simulink library "IPT_lib"  (Simulink 7.4)
settings: Solver=ode45  StartTime=0.0  StopTime=10.0  RelTol=1e-3
values from neighbouring files (symbols this model uses):
  IPTa_i_ShuntCur = mpt.Parameter    [IPT_ANALOG_CAL.m]
  IPTc_Gain_KL30 = mpt.Parameter    [IPT_ANALOG_CAL.m]
  IPTc_Gain_MSDVolt = mpt.Parameter    [IPT_ANALOG_CAL.m]
  IPTc_Gain_PCBTemp = mpt.Parameter    [IPT_ANALOG_CAL.m]
  IPTc_Gain_PosCtrVoltRef1_back = mpt.Parameter    [IPT_ANALOG_CAL.m]
  IPTc_Gain_PosCtrVoltRef1_front = mpt.Parameter    [IPT_ANALOG_CAL.m]
  IPTc_Gain_PosCtrVoltRef2_back = mpt.Parameter    [IPT_ANALOG_CAL.m]
  IPTc_Gain_PosCtrVoltRef2_front = mpt.Parameter    [IPT_ANALOG_CAL.m]
  IPTc_pct_CellInitSoc = mpt.Parameter    [IPT_INTERNAL_CAL.m]
  IPTc_t_BMUInitTemp = mpt.Parameter    [IPT_CAN_CAL.m]
  IPTc_t_MdlInitTemp = mpt.Parameter    [IPT_CAN_CAL.m]
  IPTc_t_PCBTemp_max = mpt.Parameter    [IPT_ANALOG_CAL.m]
  IPTc_t_PCBTemp_min = mpt.Parameter    [IPT_ANALOG_CAL.m]
  IPTc_v_KL30_max = mpt.Parameter    [IPT_ANALOG_CAL.m]
  IPTc_v_KL30_min = mpt.Parameter    [IPT_ANALOG_CAL.m]
  IPTc_v_MSDVolt_max = mpt.Parameter    [IPT_ANALOG_CAL.m]
  IPTc_v_MSDVolt_min = mpt.Parameter    [IPT_ANALOG_CAL.m]
  IPTc_v_PosCtrVoltRef1_back_max = mpt.Parameter    [IPT_ANALOG_CAL.m]
  IPTc_v_PosCtrVoltRef1_back_min = mpt.Parameter    [IPT_ANALOG_CAL.m]
  IPTc_v_PosCtrVoltRef1_front_max = mpt.Parameter    [IPT_ANALOG_CAL.m]
  IPTc_v_PosCtrVoltRef1_front_min = mpt.Parameter    [IPT_ANALOG_CAL.m]
  IPTc_v_PosCtrVoltRef2_back_max = mpt.Parameter    [IPT_ANALOG_CAL.m]
  IPTc_v_PosCtrVoltRef2_back_min = mpt.Parameter    [IPT_ANALOG_CAL.m]
  IPTc_v_PosCtrVoltRef2_front_max = mpt.Parameter    [IPT_ANALOG_CAL.m]
  IPTc_v_PosCtrVoltRef2_front_min = mpt.Parameter    [IPT_ANALOG_CAL.m]
  IPTf_fac_ShuntCurCorrect = mpt.Parameter    [IPT_ANALOG_CAL.m]
undefined symbols (not defined in the file or in its folder): CTC_DriveOnline_St, CTC_FastChaOnline_St, CTC_SlowChaOnline_St, IPTa_v_PCBTemp, IPTc_Gain_BMUPowSplyCur, IPTc_Gain_ShuntCur, IPTc_Gain_USample, IPTc_i_BMUPowSplyCur_max, IPTc_i_BMUPowSplyCur_min, IPTc_i_ShuntCur_max, IPTc_i_ShuntCur_min, IPTc_v_CC2_OffDnLimit, IPTc_v_CC2_OffUpLimit, IPTc_v_CC2_OnDnLimit, IPTc_v_CC2_OnUpLimit, IPTc_v_CellInitVolt, IPTc_v_SlowChalineCnctStLowLimFir, IPTc_v_SlowChalineCnctStLowLimSec, IPTc_v_SlowChalineCnctStUppLimFir, IPTc_v_SlowChalineCnctStUppLimSec, IPTc_v_SlowChalineOpenLowLim, IPTc_v_SlowChalineOpenUppLim, IPTc_v_USample_max, IPTc_v_USample_min, IPTf_t_PCBTemp, PACK_Const_BMUNumOfPack
libraries: Defined_Functionality x129
(part 3 of 3)

== system IPT_lib/IPT/ip_digitial/ChaWake ==
  HLd_adc_ChaWake : Inport  OutDataType=fixdt(1, 16)  OutScaling=2^0
  ADC to Actual Value2 : Defined_Functionality/ADC to Actual Value  SystemSampleTime=-1  gain=0.0134277  offset=0
      settings: AttributesFormatString=[GAIN=%<gain>]\n[OFFSET=%<offset>]
  LPF : Defined_Functionality/LPF  SystemSampleTime=-1  filter_gain=0.09
      settings: AttributesFormatString=[FILTER_GAIN=%<filter_gain>]
  hysteresis1 : Defined_Functionality/hysteresis  SystemSampleTime=-1  upper_limit=IPTc_v_ChaWake_HysisUpLimit  lower_limit=IPTc_v_ChaWake_HysisDnLimit
      settings: AttributesFormatString=[UPPER_LIMIT=%<upper_limit>]\n[LOWER_LIMIT=%<lower_limit>]
  signal_debug : Defined_Functionality/signal_debug  SystemSampleTime=-1  debug_switch=IPTc_dbgsw_ChaWake  debug_value=IPTc_dbgval_ChaWake
      settings: AttributesFormatString=[SWITCH=%<debug_switch>]\n[VALUE=%<debug_value>]
  IPTd_flg_ChaWake : Outport  OutDataType=fixdt(1, 16)  OutScaling=2^0
  wires:
  hysteresis1/1 -> signal_debug/1
  ADC to Actual Value2/1 -> LPF/1
  HLd_adc_ChaWake/1 -> ADC to Actual Value2/1
  signal_debug/1 -> IPTd_flg_ChaWake/1  "IPTd_flg_ChaWake"
  LPF/1 -> hysteresis1/1

== system IPT_lib/IPT/ip_digitial/HVILSt ==
  HLd_flg_HVILSt : Inport  OutDataType=fixdt(1, 16)  OutScaling=2^0
  debounce : Defined_Functionality/debounce  SystemSampleTime=-1  debounce_time=30
      settings: AttributesFormatString=[DEBOUNCE_TIME=%<debounce_time>]
  signal_debug : Defined_Functionality/signal_debug  SystemSampleTime=-1  debug_switch=IPTc_dbgsw_HVILSt  debug_value=IPTc_dbgval_HVILSt
      settings: AttributesFormatString=[SWITCH=%<debug_switch>]\n[VALUE=%<debug_value>]
  IPTd_flg_HVILSt : Outport  OutDataType=fixdt(1, 16)  OutScaling=2^0
  wires:
  debounce/1 -> signal_debug/1
  HLd_flg_HVILSt/1 -> debounce/1
  signal_debug/1 -> IPTd_flg_HVILSt/1  "IPTd_flg_HVILSt"

== system IPT_lib/IPT/ip_digitial/KL15 ==
  HLd_adc_KL15 : Inport  OutDataType=fixdt(1, 16)  OutScaling=2^0
  ADC to Actual Value3 : Defined_Functionality/ADC to Actual Value  SystemSampleTime=-1  gain=0.0134277  offset=0
      settings: AttributesFormatString=[GAIN=%<gain>]\n[OFFSET=%<offset>]
  LPF : Defined_Functionality/LPF  SystemSampleTime=-1  filter_gain=IPTc_flter_KL15
      settings: AttributesFormatString=[FILTER_GAIN=%<filter_gain>]
  hysteresis : Defined_Functionality/hysteresis  SystemSampleTime=-1  upper_limit=IPTc_v_KL15_HysisUpLimit  lower_limit=IPTc_v_KL15_HysisDnLimit
      settings: AttributesFormatString=[UPPER_LIMIT=%<upper_limit>]\n[LOWER_LIMIT=%<lower_limit>]
  signal_debug : Defined_Functionality/signal_debug  SystemSampleTime=-1  debug_switch=IPTc_dbgsw_KL15  debug_value=IPTc_dbgval_KL15
      settings: AttributesFormatString=[SWITCH=%<debug_switch>]\n[VALUE=%<debug_value>]
  IPTd_flg_KL15 : Outport  OutDataType=fixdt(1, 16)  OutScaling=2^0
  wires:
  LPF/1 -> hysteresis/1  "IPTd_v_KL15"
  ADC to Actual Value3/1 -> LPF/1
  HLd_adc_KL15/1 -> ADC to Actual Value3/1
  signal_debug/1 -> IPTd_flg_KL15/1  "IPTd_flg_KL15"
  hysteresis/1 -> signal_debug/1

== system IPT_lib/IPT/ip_digitial/ServiceSt ==
  HLd_flg_ServSt : Inport  OutDataType=fixdt(1, 16)  OutScaling=2^0
  debounce : Defined_Functionality/debounce  SystemSampleTime=-1  debounce_time=30
      settings: AttributesFormatString=[DEBOUNCE_TIME=%<debounce_time>]
  signal_debug : Defined_Functionality/signal_debug  SystemSampleTime=-1  debug_switch=IPTc_dbgsw_ServSt  debug_value=IPTc_dbgval_ServSt
      settings: AttributesFormatString=[SWITCH=%<debug_switch>]\n[VALUE=%<debug_value>]
  IPTd_flg_ServSt : Outport  OutDataType=fixdt(1, 16)  OutScaling=2^0
  wires:
  signal_debug/1 -> IPTd_flg_ServSt/1  "IPTd_flg_ServSt"
  HLd_flg_ServSt/1 -> debounce/1
  debounce/1 -> signal_debug/1

== system IPT_lib/IPT/InternalOutputOfPlatform/RestoreMdlSoc/CellSoc ==
  CellMdlIn : Inport
  Assignment : Assignment  IndexOptions=Index vector (port)  Indices=1  OutputSizes=1
  CAN to Actual Value : Defined_Functionality/CAN to Actual Value  SystemSampleTime=-1  gain=0.01  offset=0
      settings: AttributesFormatString=[GAIN=%<gain>]\n[OFFSET=%<offset>]
  Constant2 : Constant  Value=IPTc_pct_CellInitSoc
  For Iterator : ForIterator  IterationLimit=PACK_Const_MdlNumOfPack  IterationVariableDataType=int16
  Selector : Selector  InputPortWidth=PACK_Const_MdlNumOfPack  IndexOptions=Index vector (port)  Indices=[1 3]  OutputSizes=1
  CellMdlOut : Outport  DataType=single  OutDataTypeStr=single
  wires:
  Selector/1 -> CAN to Actual Value/1
  CellMdlIn/1 -> Selector/1
  For Iterator/1 -> Selector/2, Assignment/3
  Constant2/1 -> Assignment/1
  Assignment/1 -> CellMdlOut/1
  CAN to Actual Value/1 -> Assignment/2

== system IPT_lib/IPT/ip_analog/PCBTemp/Conversion ==
  ADC : Inport  OutDataType=fixdt(1, 16)  OutScaling=2^0
  ADC to Actual Value1 : Defined_Functionality/ADC to Actual Value1  SystemSampleTime=-1  offset=IPTc_Offset_PCBTemp  gain=IPTc_Gain_PCBTemp
      settings: AttributesFormatString=[OFFSET=%<offset>]\n[GAIN=%<gain>]
  Lookup Table : Lookup  InputValues=IPTa_v_PCBTemp  Table=IPTf_t_PCBTemp  OutDataType=fixdt(1, 16)  OutScaling=2^0
  Volt : Outport  OutDataType=fixdt(1, 16)  OutScaling=2^0
  wires:
  Lookup Table/1 -> Volt/1  "IPTd_t_PCBTemp_raw"
  ADC to Actual Value1/1 -> Lookup Table/1
  ADC/1 -> ADC to Actual Value1/1

== system IPT_lib/IPT/ip_can/BMU_BMS_200ms/ErrorCode ==
  In : Inport
  Assignment : Assignment  IndexOptions=Index vector (port)  Indices=1  OutputSizes=1
  Constant2 : Constant  Value=zeros(1,PACK_Const_BMUNumOfPack)  OutDataTypeMode=uint16  OutDataTypeStr=uint16
  For Iterator : ForIterator  IterationLimit=PACK_Const_BMUNumOfPack  IterationVariableDataType=int16
  Selector : Selector  InputPortWidth=PACK_Const_BMUNumOfPack  IndexOptions=Index vector (port)  Indices=[1 3]  OutputSizes=1
  Out : Outport
  wires:
  Assignment/1 -> Out/1
  Constant2/1 -> Assignment/1
  For Iterator/1 -> Assignment/3, Selector/2
  In/1 -> Selector/1
  Selector/1 -> Assignment/2

== system IPT_lib/IPT/ip_can/BMU_BMS_200ms/NmStatus ==
  In : Inport
  Assignment : Assignment  IndexOptions=Index vector (port)  Indices=1  OutputSizes=1
  Constant2 : Constant  Value=zeros(1,PACK_Const_BMUNumOfPack)  OutDataTypeMode=uint8  OutDataTypeStr=uint8
  For Iterator : ForIterator  IterationLimit=PACK_Const_BMUNumOfPack  IterationVariableDataType=int16
  Selector : Selector  InputPortWidth=PACK_Const_BMUNumOfPack  IndexOptions=Index vector (port)  Indices=[1 3]  OutputSizes=1
  Out : Outport
  wires:
  Selector/1 -> Assignment/2
  In/1 -> Selector/1
  For Iterator/1 -> Selector/2, Assignment/3
  Constant2/1 -> Assignment/1
  Assignment/1 -> Out/1

== system IPT_lib/IPT/ip_can/BMU_BMS_200ms/NodeStatus ==
  In : Inport
  Assignment : Assignment  IndexOptions=Index vector (port)  Indices=1  OutputSizes=1
  Constant2 : Constant  Value=zeros(1,PACK_Const_BMUNumOfPack)  OutDataTypeMode=uint8  OutDataTypeStr=uint8
  For Iterator : ForIterator  IterationLimit=PACK_Const_BMUNumOfPack  IterationVariableDataType=int16
  Selector : Selector  InputPortWidth=PACK_Const_BMUNumOfPack  IndexOptions=Index vector (port)  Indices=[1 3]  OutputSizes=1
  Out : Outport
  wires:
  Assignment/1 -> Out/1
  Constant2/1 -> Assignment/1
  For Iterator/1 -> Assignment/3, Selector/2
  In/1 -> Selector/1
  Selector/1 -> Assignment/2

== system IPT_lib/IPT/ip_can/BMU_BMS_300ms/CellVolt ==
  In : Inport
  Assignment : Assignment  IndexOptions=Index vector (port)  Indices=1  OutputSizes=1
  CAN to Actual Value : Defined_Functionality/CAN to Actual Value  SystemSampleTime=-1  gain=0.001  offset=0
      settings: AttributesFormatString=[GAIN=%<gain>]\n[OFFSET=%<offset>]
  Constant2 : Constant  Value=IPTc_v_CellInitVolt
  For Iterator : ForIterator  IterationLimit=PACK_Const_CellNumOfPack  IterationVariableDataType=int16
  LPF : Defined_Functionality/LPF  SystemSampleTime=-1  filter_gain=IPTc_flter_CellVolt
      settings: AttributesFormatString=[FILTER_GAIN=%<filter_gain>]
  Selector : Selector  InputPortWidth=PACK_Const_CellNumOfPack  IndexOptions=Index vector (port)  Indices=[1 3]  OutputSizes=1
  Out : Outport
  wires:
  LPF/1 -> Assignment/2
  Selector/1 -> CAN to Actual Value/1
  In/1 -> Selector/1
  For Iterator/1 -> Assignment/3, Selector/2
  Constant2/1 -> Assignment/1
  Assignment/1 -> Out/1
  CAN to Actual Value/1 -> LPF/1

== system IPT_lib/IPT/ip_can/BMU_BMS_500ms/BMUTemp ==
  In : Inport
  Assignment : Assignment  IndexOptions=Index vector (port)  Indices=1  OutputSizes=1
  CAN to Actual Value : Defined_Functionality/CAN to Actual Value  SystemSampleTime=-1  gain=1  offset=-40
      settings: AttributesFormatString=[GAIN=%<gain>]\n[OFFSET=%<offset>]
  Constant2 : Constant  Value=IPTc_t_BMUInitTemp  OutDataTypeMode=single  OutDataTypeStr=single
  For Iterator : ForIterator  IterationLimit=PACK_Const_BMUTempSnrNumOfPack  IterationVariableDataType=int16
  LPF : Defined_Functionality/LPF  SystemSampleTime=-1  filter_gain=IPTc_flter_BMUTemp
      settings: AttributesFormatString=[FILTER_GAIN=%<filter_gain>]
  Selector : Selector  InputPortWidth=PACK_Const_BMUTempSnrNumOfPack  IndexOptions=Index vector (port)  Indices=[1 3]  OutputSizes=1
  Out : Outport
  wires:
  LPF/1 -> Assignment/2
  In/1 -> Selector/1
  For Iterator/1 -> Selector/2, Assignment/3
  Constant2/1 -> Assignment/1
  Assignment/1 -> Out/1
  Selector/1 -> CAN to Actual Value/1
  CAN to Actual Value/1 -> LPF/1

== system IPT_lib/IPT/ip_can/BMU_BMS_500ms/MdlTemp ==
  In : Inport
  Assignment : Assignment  IndexOptions=Index vector (port)  Indices=1  OutputSizes=1
  CAN to Actual Value : Defined_Functionality/CAN to Actual Value  SystemSampleTime=-1  gain=0.125  offset=-40
      settings: AttributesFormatString=[GAIN=%<gain>]\n[OFFSET=%<offset>]
  Constant2 : Constant  Value=IPTc_t_MdlInitTemp  OutDataTypeMode=single  OutDataTypeStr=single
  For Iterator : ForIterator  IterationLimit=PACK_Const_MdlTempSnrNumOfPack  IterationVariableDataType=int16
  LPF : Defined_Functionality/LPF  SystemSampleTime=-1  filter_gain=IPTc_flter_MdlTemp
      settings: AttributesFormatString=[FILTER_GAIN=%<filter_gain>]
  Selector : Selector  InputPortWidth=PACK_Const_MdlTempSnrNumOfPack  IndexOptions=Index vector (port)  Indices=[1 3]  OutputSizes=1
  Out : Outport
  wires:
  LPF/1 -> Assignment/2
  CAN to Actual Value/1 -> LPF/1
  Selector/1 -> CAN to Actual Value/1
  Assignment/1 -> Out/1
  Constant2/1 -> Assignment/1
  For Iterator/1 -> Assignment/3, Selector/2
  In/1 -> Selector/1

== system IPT_lib/IPT/ip_can/Diagnositc_Enabling/CAN_Bus_Monitoring ==
  HLd_flg_CANBusOff : Inport
  Gain : Gain  OutDataTypeStr=Inherit: Inherit via back propagation
  debounce : Defined_Functionality/debounce  SystemSampleTime=-1  debounce_time=IPTc_tm_CANBusOffDeb
      settings: AttributesFormatString=[DEBOUNCE_TIME=%<debounce_time>]
  IPTd_iflt_CANBusOff_fault : Outport
  IPTd_cflt_CANBusOff_fault : Outport  Port=2
  wires:
  debounce/1 -> IPTd_cflt_CANBusOff_fault/1
  Gain/1 -> debounce/1, IPTd_iflt_CANBusOff_fault/1
  HLd_flg_CANBusOff/1 -> Gain/1

== system IPT_lib/IPT/ip_can/Diagnositc_Enabling/CAN_Diag_Enabling ==
  IPTd_iflt_CANBusOff_fault : Inport
  IPTd_cflt_CANBusOff_fault : Inport  Port=2
  IPTd_flg_KL15 : Inport  Port=3
  Logical Operator : Logic  Inputs=3  AllPortsSameDT=off  OutDataTypeMode=boolean  LogicDataType=fixdt(0, 8)  OutDataTypeStr=boolean
  Logical Operator2 : Logic  Operator=NOT  Inputs=1  AllPortsSameDT=off  OutDataTypeMode=boolean  OutDataTypeStr=boolean
  Logical Operator3 : Logic  Operator=NOT  Inputs=1  AllPortsSameDT=off  OutDataTypeMode=boolean  OutDataTypeStr=boolean
  rising_delay : Defined_Functionality/rising_delay  SystemSampleTime=-1  delay_time=500
      settings: AttributesFormatString=[DELAY_TIME=%<delay_time>]
  signal_debug : Defined_Functionality/signal_debug  SystemSampleTime=-1  debug_switch=IPTc_dbgsw_CANDiagEnable  debug_value=IPTc_dbgval_CANDiagEnable
      settings: AttributesFormatString=[SWITCH=%<debug_switch>]\n[VALUE=%<debug_value>]
  IPTd_flg_CANDiagEnable : Outport
  wires:
  signal_debug/1 -> IPTd_flg_CANDiagEnable/1  "IPTd_flg_CANDiagEnable"
  Logical Operator/1 -> signal_debug/1
  Logical Operator3/1 -> Logical Operator/2
  IPTd_cflt_CANBusOff_fault/1 -> Logical Operator3/1
  rising_delay/1 -> Logical Operator/3
  Logical Operator2/1 -> Logical Operator/1
  IPTd_flg_KL15/1 -> rising_delay/1
  IPTd_iflt_CANBusOff_fault/1 -> Logical Operator2/1

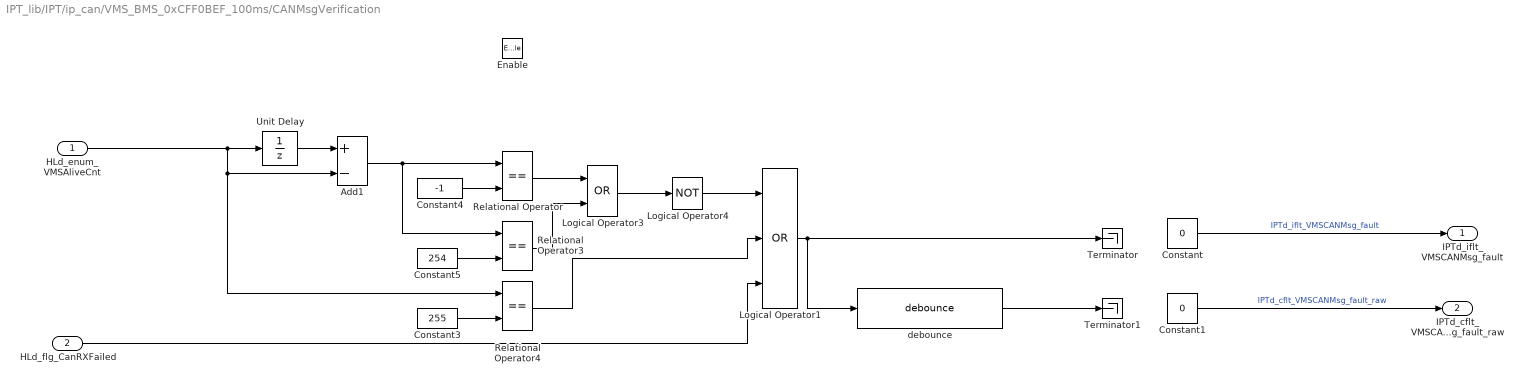
== system IPT_lib/IPT/ip_can/VMS_BMS_0xCFF0BEF_100ms/CANMsgVerification ==
  HLd_enum_VMSAliveCnt : Inport
  HLd_flg_CanRXFailed : Inport  Port=2  OutDataType=fixdt(1, 16)  OutScaling=2^0
  Enable : EnablePort
  Add1 : Sum  Inputs=+-  OutDataTypeMode=int16  OutDataTypeStr=int16
  Constant : Constant  Value=0  OutDataTypeMode=boolean  OutDataType=fixdt(1, 16)  OutScaling=2^0  OutDataTypeStr=boolean
  Constant1 : Constant  Value=0  OutDataTypeMode=boolean  OutDataType=fixdt(1, 16)  OutScaling=2^0  OutDataTypeStr=boolean
  Constant3 : Constant  Value=255  OutDataTypeMode=uint8  OutDataTypeStr=uint8
  Constant4 : Constant  Value=-1  OutDataTypeMode=int8  OutDataTypeStr=int8
  Constant5 : Constant  Value=254  OutDataTypeMode=uint8  OutDataTypeStr=uint8
  Logical Operator1 : Logic  Operator=OR  Inputs=3  AllPortsSameDT=off  OutDataTypeMode=boolean  LogicDataType=fixdt(0, 8)  OutDataTypeStr=boolean
  Logical Operator3 : Logic  Operator=OR  AllPortsSameDT=off  OutDataTypeMode=boolean  LogicDataType=fixdt(0, 8)  OutDataTypeStr=boolean
  Logical Operator4 : Logic  Operator=NOT  AllPortsSameDT=off  OutDataTypeMode=boolean  LogicDataType=fixdt(0, 8)  OutDataTypeStr=boolean
  Relational Operator : RelationalOperator  Operator===  LogicOutDataTypeMode=boolean  OutDataTypeStr=boolean
  Relational Operator3 : RelationalOperator  Operator===  LogicOutDataTypeMode=boolean  OutDataTypeStr=boolean
  Relational Operator4 : RelationalOperator  Operator===  LogicOutDataTypeMode=boolean  OutDataTypeStr=boolean
  Terminator : Terminator
  Terminator1 : Terminator
  Unit Delay : UnitDelay  SampleTime=-1
  debounce : Defined_Functionality/debounce  SystemSampleTime=-1  debounce_time=IPTc_tm_VMSCanFltDeb
      settings: AttributesFormatString=[DEBOUNCE_TIME=%<debounce_time>]
  IPTd_iflt_VMSCANMsg_fault : Outport  InitialOutput=0
  IPTd_cflt_VMSCANMsg_fault_raw : Outport  Port=2  InitialOutput=0
  wires:
  Constant1/1 -> IPTd_cflt_VMSCANMsg_fault_raw/1  "IPTd_cflt_VMSCANMsg_fault_raw"
  Constant/1 -> IPTd_iflt_VMSCANMsg_fault/1  "IPTd_iflt_VMSCANMsg_fault"
  Logical Operator3/1 -> Logical Operator4/1
  Relational Operator4/1 -> Logical Operator1/2
  Constant3/1 -> Relational Operator4/2
  Relational Operator3/1 -> Logical Operator3/2
  Relational Operator/1 -> Logical Operator3/1
  Add1/1 -> Relational Operator3/1, Relational Operator/1
  Unit Delay/1 -> Add1/1
  Constant4/1 -> Relational Operator/2
  Constant5/1 -> Relational Operator3/2
  HLd_enum_VMSAliveCnt/1 -> Relational Operator4/1, Add1/2, Unit Delay/1
  Logical Operator4/1 -> Logical Operator1/1
  Logical Operator1/1 -> Terminator/1, debounce/1
  HLd_flg_CanRXFailed/1 -> Logical Operator1/3
  debounce/1 -> Terminator1/1

== system IPT_lib/IPT/ip_can/VMS_BMS_0xCFF0BEF_100ms/HVCnctCmd ==
  HLd_flg_VehHVCnctCmd : Inport
  IPTd_iflt_VMSCANMsg_fault : Inport  Port=2
  IPTd_cflt_VMSCANMsg_fault_raw : Inport  Port=3
  Constant : Constant  Value=0  OutDataTypeMode=boolean  OutDataType=fixdt(1, 16)  OutScaling=2^0  OutDataTypeStr=boolean
  Logical Operator : Logic  Operator=NOT  AllPortsSameDT=off  OutDataTypeMode=boolean  LogicDataType=fixdt(0, 8)  OutDataTypeStr=boolean
  Switch : Switch  Criteria=u2 > Threshold  OutDataType=fixdt(1, 16)  OutScaling=2^0
  Switch2 : Switch  Criteria=u2 > Threshold  OutDataType=fixdt(1, 16)  OutScaling=2^0
  Unit Delay : UnitDelay  SampleTime=-1
  signal_debug : Defined_Functionality/signal_debug  SystemSampleTime=-1  debug_switch=IPTc_dbgsw_VehHVCnctCmd  debug_value=IPTc_dbgval_VehHVCnctCmd
      settings: AttributesFormatString=[SWITCH=%<debug_switch>]\n[VALUE=%<debug_value>]
  IPTd_flg_VehHVCnctCmd : Outport
  wires:
  IPTd_iflt_VMSCANMsg_fault/1 -> Switch2/2
  IPTd_cflt_VMSCANMsg_fault_raw/1 -> Logical Operator/1
  HLd_flg_VehHVCnctCmd/1 -> [HLd_flg_VehHVCnctCmd], Unit Delay/1
  Constant/1 -> Switch/3
  Switch2/1 -> Switch/1
  [HLd_flg_VehHVCnctCmd] -> Switch2/3
  Unit Delay/1 -> Switch2/1
  Logical Operator/1 -> Switch/2
  Switch/1 -> signal_debug/1
  signal_debug/1 -> IPTd_flg_VehHVCnctCmd/1  "IPTd_flg_VehHVCnctCmd"

== system IPT_lib/IPT/ip_can/VMS_BMS_0xCFF0BEF_100ms/KeySt ==
  HLd_enum_KeySt : Inport
  IPTd_cflt_VMSCANMsg_fault_raw : Inport  Port=2
  Constant : Constant  Value=0  OutDataTypeMode=uint8  OutDataType=fixdt(1, 16)  OutScaling=2^0  OutDataTypeStr=uint8
  Constant1 : Constant  Value=3  OutDataTypeMode=uint8  OutDataType=fixdt(1, 16)  OutScaling=2^0  OutDataTypeStr=uint8
  Gain : Gain  ParameterDataType=fixdt(1, 16)  ParameterScaling=2^0  OutDataType=fixdt(1, 16)  OutScaling=2^0  OutDataTypeStr=Inherit: Same as input
  Logical Operator : Logic  Operator=NOT  AllPortsSameDT=off  OutDataTypeMode=boolean  LogicDataType=fixdt(0, 8)  OutDataTypeStr=boolean
  Logical Operator2 : Logic  Operator=OR  AllPortsSameDT=off  OutDataTypeMode=boolean  LogicDataType=fixdt(0, 8)  OutDataTypeStr=boolean
  Relational Operator : RelationalOperator  Operator=>  LogicOutDataTypeMode=boolean  LogicDataType=fixdt(0, 8)  OutDataTypeStr=boolean
  Switch : Switch  Criteria=u2 > Threshold  OutDataType=fixdt(1, 16)  OutScaling=2^0
  Switch2 : Switch  Criteria=u2 > Threshold  OutDataType=fixdt(1, 16)  OutScaling=2^0
  Unit Delay : UnitDelay  SampleTime=-1
  debounce : Defined_Functionality/debounce  SystemSampleTime=-1  debounce_time=IPTc_tm_VMSCanFltDeb
      settings: AttributesFormatString=[DEBOUNCE_TIME=%<debounce_time>]
  signal_debug : Defined_Functionality/signal_debug  SystemSampleTime=-1  debug_switch=0  debug_value=1
      settings: AttributesFormatString=[SWITCH=%<debug_switch>]\n[VALUE=%<debug_value>]
  IPTd_enum_KeySt : Outport
  wires:
  Gain/1 -> [IPTd_enum_KeyStRaw]
  Relational Operator/1 -> Logical Operator2/1
  Logical Operator2/1 -> Switch2/2, debounce/1  "IPTd_iflt_CANBus"
  Constant1/1 -> Relational Operator/2
  IPTd_cflt_VMSCANMsg_fault_raw/1 -> Logical Operator2/2
  [IPTd_enum_KeyStRaw] -> Switch2/3
  debounce/1 -> Logical Operator/1
  HLd_enum_KeySt/1 -> Gain/1, Unit Delay/1, Relational Operator/1
  Switch/1 -> signal_debug/1
  Unit Delay/1 -> Switch2/1
  Switch2/1 -> Switch/1
  Constant/1 -> Switch/3
  Logical Operator/1 -> Switch/2
  signal_debug/1 -> IPTd_enum_KeySt/1  "IPTd_enum_KeySt"

== system IPT_lib/IPT/ip_can/VMS_BMS_0xCFF0BEF_100ms/VMSChaAllowed ==
  HLd_flg_VMSChaAllowed : Inport  DataType=boolean  OutDataTypeStr=boolean
  IPTd_iflt_CANMsg_fault : Inport  Port=2
  IPTd_cflt_VMSCANMsg_fault_raw : Inport  Port=3
  Constant : Constant  Value=0  OutDataTypeMode=boolean  OutDataType=fixdt(1, 16)  OutScaling=2^0  OutDataTypeStr=boolean
  Logical Operator : Logic  Operator=NOT  AllPortsSameDT=off  OutDataTypeMode=boolean  LogicDataType=fixdt(0, 8)  OutDataTypeStr=boolean
  Switch : Switch  Criteria=u2 > Threshold  OutDataType=fixdt(1, 16)  OutScaling=2^0
  Switch2 : Switch  Criteria=u2 > Threshold  OutDataType=fixdt(1, 16)  OutScaling=2^0
  Unit Delay1 : UnitDelay  SampleTime=-1
  debounce : Defined_Functionality/debounce  SystemSampleTime=-1  debounce_time=IPTc_tm_VMSChaAllowedDeb
      settings: AttributesFormatString=[DEBOUNCE_TIME=%<debounce_time>]
  signal_debug1 : Defined_Functionality/signal_debug  SystemSampleTime=-1  debug_switch=IPTc_dbgsw_VMSChaAllowed  debug_value=IPTc_dbgval_VMSChaAllowed
      settings: AttributesFormatString=[SWITCH=%<debug_switch>]\n[VALUE=%<debug_value>]
  IPTd_flg_VMSChaAllowed : Outport
  wires:
  debounce/1 -> signal_debug1/1
  IPTd_iflt_CANMsg_fault/1 -> Switch2/2
  IPTd_cflt_VMSCANMsg_fault_raw/1 -> Logical Operator/1
  HLd_flg_VMSChaAllowed/1 -> [HLd_flg_VMSChaAllowed], Unit Delay1/1
  Unit Delay1/1 -> Switch2/1
  [HLd_flg_VMSChaAllowed] -> Switch2/3
  Switch2/1 -> Switch/1
  Logical Operator/1 -> Switch/2
  Switch/1 -> debounce/1
  Constant/1 -> Switch/3
  signal_debug1/1 -> IPTd_flg_VMSChaAllowed/1  "IPTd_flg_VMSChaAllowed"

== system IPT_lib/IPT/ip_can/VMS_BMS_0xCFF0BEF_100ms/VMSChaStopCmd ==
  HLd_flg_VMSChaStopCmd : Inport  DataType=boolean  OutDataTypeStr=boolean
  IPTd_iflt_CANMsg_fault : Inport  Port=2
  IPTd_cflt_VMSCANMsg_fault_raw : Inport  Port=3
  Constant : Constant  OutDataTypeMode=boolean  OutDataType=fixdt(1, 16)  OutScaling=2^0  OutDataTypeStr=boolean
  Logical Operator : Logic  Operator=NOT  AllPortsSameDT=off  OutDataTypeMode=boolean  LogicDataType=fixdt(0, 8)  OutDataTypeStr=boolean
  Switch : Switch  Criteria=u2 > Threshold  OutDataType=fixdt(1, 16)  OutScaling=2^0
  Switch1 : Switch  Criteria=u2 > Threshold  OutDataType=fixdt(1, 16)  OutScaling=2^0
  Unit Delay : UnitDelay  SampleTime=-1
  debounce : Defined_Functionality/debounce  SystemSampleTime=-1  debounce_time=IPTc_tm_VMSChaStopCmdDeb
      settings: AttributesFormatString=[DEBOUNCE_TIME=%<debounce_time>]
  signal_debug : Defined_Functionality/signal_debug  SystemSampleTime=-1  debug_switch=IPTc_dbgsw_VMSChaStopCmd  debug_value=IPTc_dbgval_VMSChaStopCmd
      settings: AttributesFormatString=[SWITCH=%<debug_switch>]\n[VALUE=%<debug_value>]
  IPTd_flg_VMSChaStopCmd : Outport
  wires:
  HLd_flg_VMSChaStopCmd/1 -> [HLd_flg_VMSChaStopCmd], Unit Delay/1
  IPTd_iflt_CANMsg_fault/1 -> Switch1/2
  debounce/1 -> signal_debug/1
  [HLd_flg_VMSChaStopCmd] -> Switch1/3
  Switch1/1 -> Switch/1
  Unit Delay/1 -> Switch1/1
  Constant/1 -> Switch/3
  Logical Operator/1 -> Switch/2
  Switch/1 -> debounce/1
  IPTd_cflt_VMSCANMsg_fault_raw/1 -> Logical Operator/1
  signal_debug/1 -> IPTd_flg_VMSChaStopCmd/1  "IPTd_flg_VMSChaStopCmd"

== system IPT_lib/IPT/ip_can/VMS_BMS_0xCFF0BEF_100ms/VehShutBCUCmd ==
  HLd_flg_VehShutBCUCmd : Inport
  IPTd_iflt_CANMsg_fault : Inport  Port=2
  IPTd_cflt_VMSCANMsg_fault_raw : Inport  Port=3
  Constant : Constant  Value=0  OutDataTypeMode=boolean  OutDataType=fixdt(1, 16)  OutScaling=2^0  OutDataTypeStr=boolean
  Logical Operator : Logic  Operator=NOT  AllPortsSameDT=off  OutDataTypeMode=boolean  LogicDataType=fixdt(0, 8)  OutDataTypeStr=boolean
  Switch : Switch  Criteria=u2 > Threshold  OutDataType=fixdt(1, 16)  OutScaling=2^0
  Switch1 : Switch  Criteria=u2 > Threshold  OutDataType=fixdt(1, 16)  OutScaling=2^0
  Unit Delay1 : UnitDelay  SampleTime=-1
  debounce : Defined_Functionality/debounce  SystemSampleTime=-1  debounce_time=IPTc_tm_VehShutBCUCmdDeb
      settings: AttributesFormatString=[DEBOUNCE_TIME=%<debounce_time>]
  signal_debug : Defined_Functionality/signal_debug  SystemSampleTime=-1  debug_switch=IPTc_dbgsw_VehShutBCUCmd  debug_value=IPTc_dbgval_VehShutBCUCmd
      settings: AttributesFormatString=[SWITCH=%<debug_switch>]\n[VALUE=%<debug_value>]
  IPTd_flg_VehShutBCUCmd : Outport
  wires:
  HLd_flg_VehShutBCUCmd/1 -> [HLd_flg_VehShutBCUCmd], Unit Delay1/1
  IPTd_cflt_VMSCANMsg_fault_raw/1 -> Logical Operator/1
  IPTd_iflt_CANMsg_fault/1 -> Switch1/2
  debounce/1 -> signal_debug/1
  Unit Delay1/1 -> Switch1/1
  [HLd_flg_VehShutBCUCmd] -> Switch1/3
  Switch1/1 -> Switch/1
  Constant/1 -> Switch/3
  Logical Operator/1 -> Switch/2
  Switch/1 -> debounce/1
  signal_debug/1 -> IPTd_flg_VehShutBCUCmd/1  "IPTd_flg_VehShutBCUCmd"

== stateflow chart IPT/ip_can/ip_can_scheduler ==
  state trigger_300ms [parallel]
    settings: executionOrder=3
    state COUNTER
      (junction 12) -> (junction 11) : {out3=counter3;counter3+=1;}
      trigger_300ms.COUNTER -> (junction 12) [order 1]
      (default) -> (junction 12) : {counter3=1;}
    trigger_300ms.COUNTER -> (junction 14) [order 1] : [out3>=30]
    (junction 13) -> trigger_300ms.COUNTER
    (junction 14) -> (junction 13) : {trigger_BMU_300ms;}
    (default) -> trigger_300ms.COUNTER : {trigger_BMU_300ms;}
  state trigger_100ms [parallel]
    settings: executionOrder=1
    state COUNTER
      (default) -> (junction 18) : {counter1=1;}
      trigger_100ms.COUNTER -> (junction 18) [order 1]
      (junction 18) -> (junction 17) : {out1=counter1;counter1+=1;}
    (junction 15) -> trigger_100ms.COUNTER
    trigger_100ms.COUNTER -> (junction 16) [order 1] : [out1>=10]
    (junction 16) -> (junction 15) : {trigger_0xCFF0BEF_100ms;}
    (default) -> trigger_100ms.COUNTER : {trigger_0xCFF0BEF_100ms;}
  state trigger_200ms [parallel]
    settings: executionOrder=2
    state COUNTER
      (default) -> (junction 21) : {counter2=1;}
      trigger_200ms.COUNTER -> (junction 21) [order 1]
      (junction 21) -> (junction 22) : {out2=counter2;counter2+=1;}
    (junction 19) -> trigger_200ms.COUNTER
    trigger_200ms.COUNTER -> (junction 20) [order 1] : [out2>=20]
    (junction 20) -> (junction 19) : {trigger_BMU_200ms;}
    (default) -> trigger_200ms.COUNTER : {trigger_BMU_200ms;}
  state trigger_500ms [parallel]
    settings: executionOrder=4
    state COUNTER
      (default) -> (junction 25) : {counter4=1;}
      trigger_500ms.COUNTER -> (junction 25) [order 1]
      (junction 25) -> (junction 26) : {out4=counter4;counter4+=1;}
    (default) -> trigger_500ms.COUNTER : {trigger_0x18FF47F8_500ms;
        | trigger_BMU_500ms;}
    (junction 23) -> trigger_500ms.COUNTER
    trigger_500ms.COUNTER -> (junction 24) [order 1] : [out4>=50]
    (junction 24) -> (junction 23) : {trigger_0x18FF47F8_500ms;
        | trigger_BMU_500ms;}
  (default) -> trigger_100ms
  data: counter1 local uint8; counter3 local uint8; out2 local uint8; out3 local uint8; out1 local uint8; counter2 local uint8; out4 local uint8; counter4 local uint8
  events: event local EITHER_EDGE_EVENT; event local EITHER_EDGE_EVENT; event local EITHER_EDGE_EVENT; trigger_0xCFF0BEF_100ms output FUNCTION_CALL_EVENT; trigger_BMU_200ms output FUNCTION_CALL_EVENT; trigger_BMU_300ms output FUNCTION_CALL_EVENT; trigger_0x18FF47F8_500ms output FUNCTION_CALL_EVENT; trigger_BMU_500ms output FUNCTION_CALL_EVENT
